simulink model "Project_LQR_MODEL_SIL"  (R2023b)
settings: Solver=VariableStepAuto  StartTime=0.0  StopTime=5  MaxStep=0.001  RelTol=1e-3
undefined symbols (not defined in the file or in its folder): A, B, C, D, k
libraries: simulink_extras x2
settings Model: Creator=AHMED MOHSEN  LastModifiedBy=AHMED MOHSEN

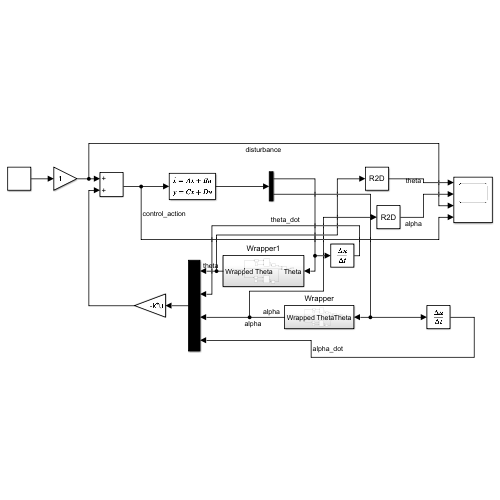
[thumbnail: Simulink's stored preview of the top-level diagram]
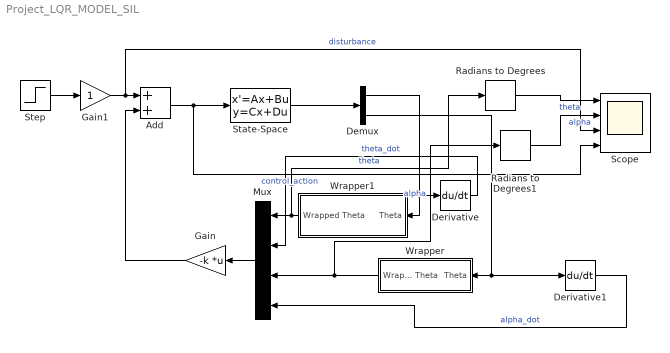
== system Project_LQR_MODEL_SIL ==
  Add : Sum
  Demux : Demux  Outputs=2
  Derivative : Derivative
  Derivative1 : Derivative
  Gain : Gain  Gain=-k  Multiplication=Matrix(K*u)
  Gain1 : Gain
  Mux : Mux
  Radians to Degrees : simulink_extras/Transformations/Radians to Degrees
  Radians to Degrees1 : simulink_extras/Transformations/Radians to Degrees
  Scope : Scope  NumInputPorts=4
  State-Space : StateSpace  A=A  B=B  C=C  D=D  InitialCondition=0
  Step : Step  SampleTime=0
  Wrapper : Subsystem
  Wrapper1 : Subsystem
  wires:
  State-Space/1 -> Demux/1
  Demux/1 -> Derivative/1, Wrapper1/1(Theta)
  Demux/2 -> Wrapper/1(Theta), Derivative1/1
  Derivative/1 -> Mux/2  "theta_dot"
  Derivative1/1 -> Mux/4  "alpha_dot"
  Wrapper/1(Wrapped Theta) -> Mux/3, Radians to Degrees1/1  "alpha"
  Wrapper1/1(Wrapped Theta) -> Radians to Degrees/1, Mux/1  "theta"
  Mux/1 -> Gain/1
  Gain/1 -> Add/2
  Add/1 -> Scope/4, State-Space/1  "control_action"
  Step/1 -> Gain1/1
  Radians to Degrees/1 -> Scope/1  "theta"
  Radians to Degrees1/1 -> Scope/2  "alpha"
  Gain1/1 -> Add/1, Scope/3  "disturbance"

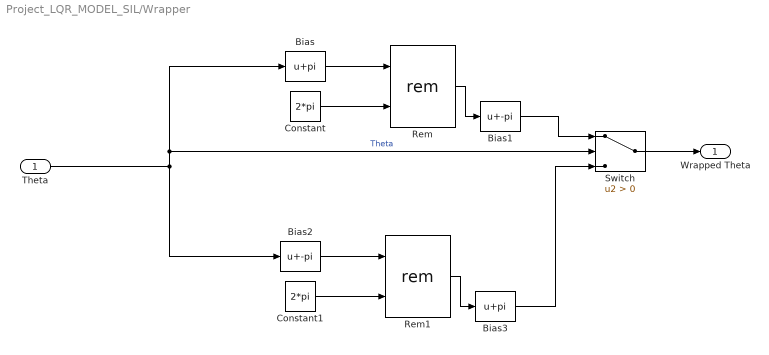
== system Project_LQR_MODEL_SIL/Wrapper ==
  Theta : Inport
  Bias : Bias  Bias=pi  SaturateOnIntegerOverflow=off
  Bias1 : Bias  Bias=-pi  SaturateOnIntegerOverflow=off
  Bias2 : Bias  Bias=-pi  SaturateOnIntegerOverflow=off
  Bias3 : Bias  Bias=pi  SaturateOnIntegerOverflow=off
  Constant : Constant  Value=2*pi
  Constant1 : Constant  Value=2*pi
  Rem : Math  Operator=rem
  Rem1 : Math  Operator=rem
  Switch : Switch  Criteria=u2 > Threshold  SaturateOnIntegerOverflow=off  InputSameDT=off
  Wrapped Theta : Outport
  wires:
  Theta/1 -> Bias2/1, Bias/1, Switch/2  "Theta"
  Bias/1 -> Rem/1
  Constant/1 -> Rem/2
  Rem/1 -> Bias1/1
  Bias1/1 -> Switch/1
  Constant1/1 -> Rem1/2
  Rem1/1 -> Bias3/1
  Bias2/1 -> Rem1/1
  Bias3/1 -> Switch/3
  Switch/1 -> Wrapped Theta/1

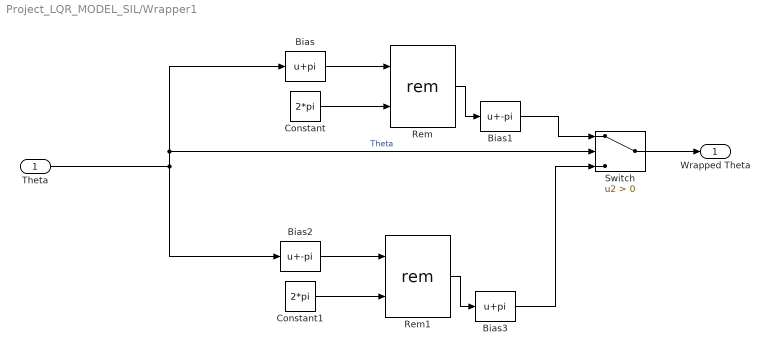
== system Project_LQR_MODEL_SIL/Wrapper1 ==
  Theta : Inport
  Bias : Bias  Bias=pi  SaturateOnIntegerOverflow=off
  Bias1 : Bias  Bias=-pi  SaturateOnIntegerOverflow=off
  Bias2 : Bias  Bias=-pi  SaturateOnIntegerOverflow=off
  Bias3 : Bias  Bias=pi  SaturateOnIntegerOverflow=off
  Constant : Constant  Value=2*pi
  Constant1 : Constant  Value=2*pi
  Rem : Math  Operator=rem
  Rem1 : Math  Operator=rem
  Switch : Switch  Criteria=u2 > Threshold  SaturateOnIntegerOverflow=off  InputSameDT=off
  Wrapped Theta : Outport
  wires:
  Theta/1 -> Bias2/1, Bias/1, Switch/2  "Theta"
  Bias/1 -> Rem/1
  Constant/1 -> Rem/2
  Rem/1 -> Bias1/1
  Bias1/1 -> Switch/1
  Constant1/1 -> Rem1/2
  Rem1/1 -> Bias3/1
  Bias2/1 -> Rem1/1
  Bias3/1 -> Switch/3
  Switch/1 -> Wrapped Theta/1
